simulink model "model"  (R2025b)
settings: Solver=FixedStepDiscrete  StartTime=0.0  StopTime=620  FixedStep=deltaT  RelTol=1e-3
values from neighbouring files (symbols this model uses):
  DegreeToRadian = pi/180    (= 0.0174532925199)    [main8.m]    (also in modelRunner.m)
  g = 9.81    [main8.m]    (also in modelRunner.m)
  Mass = 1.3    [main8.m]    (also in modelRunner.m)
  R_phi = place(A_phi, B_phi, poles_phi)    [main8.m]    (also in modelRunner.m)
  R_psi = place(A_psi, B_psi, poles_psi)    [main8.m]    (also in modelRunner.m)
  R_theta = place(A_theta, B_theta, poles_theta)    [main8.m]    (also in modelRunner.m)
  R_x = place(A_x, B_x, poles_x)    [main8.m]    (also in modelRunner.m)
  R_y = place(A_y, B_y, poles_y)    [main8.m]    (also in modelRunner.m)
  R_z = place(A_z, B_z, poles_z)    [main8.m]    (also in modelRunner.m)
  trajectory_data = TrajectorySetup()    [modelRunner.m]
settings Model: Creator=kuba  LastModifiedBy=kuba

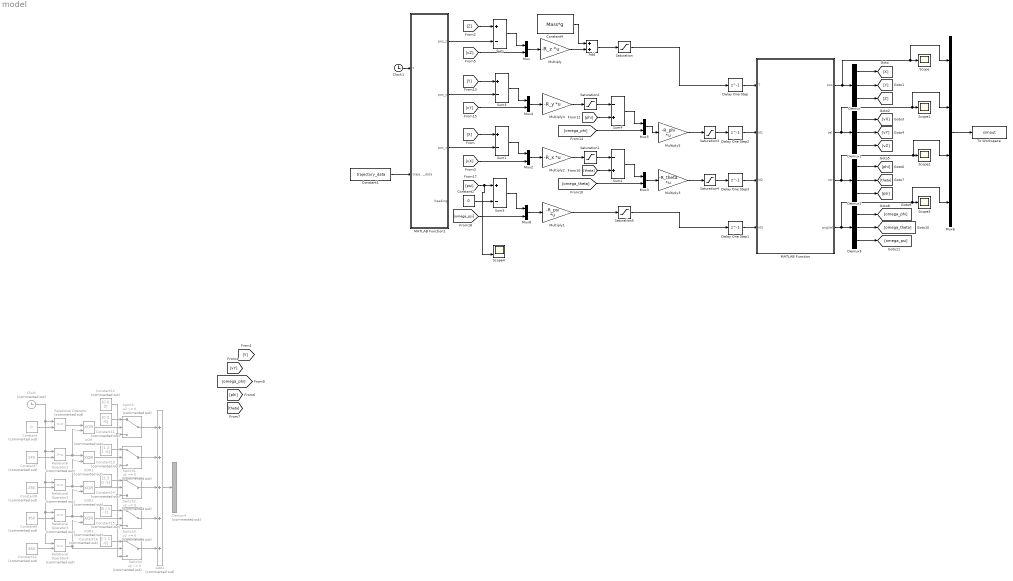
== system model ==
  Add : Sum
  Add1 : Sum  Commented=on  Inputs=+++++
  Clock : Clock  Commented=on
  Clock1 : Clock
  Constant : Constant  Commented=on  Value=0
  Constant1 : Constant  Value=trajectory_data  OutDataTypeStr=Bus: trajectory_data_bus
  Constant10 : Constant  Commented=on  Value=480
  Constant11 : Constant  Commented=on  Value=[0 0 -6]
  Constant12 : Constant  Commented=on  Value=[0 0 0]
  Constant13 : Constant  Commented=on  Value=[1.2 1 -6]
  Constant14 : Constant  Commented=on  Value=[1.5 0 -5]
  Constant15 : Constant  Commented=on  Value=[0 1.5 -7]
  Constant16 : Constant  Commented=on  Value=[-1 1 -6]
  Constant2 : Constant  Value=0
  Constant4 : Constant  Value=Mass*g
  Constant7 : Constant  Commented=on  Value=140
  Constant8 : Constant  Commented=on  Value=280
  Constant9 : Constant  Commented=on  Value=360
  Delay One Step{,1..3} (4 alike) : Delay  DelayLength=1
  Demux{,1..3} (4 alike) : Demux  Outputs=3
  Demux4 : Demux  Commented=on  Outputs=3
  MATLAB Function : MATLAB Function  TreatAsAtomicUnit=on
  MATLAB Function1 : MATLAB Function  TreatAsAtomicUnit=on
  Multiply : Gain  Gain=-R_z  Multiplication=Matrix(K*u)
  Multiply1 : Gain  Gain=-R_psi  Multiplication=Matrix(K*u)
  Multiply2 : Gain  Gain=-R_x  Multiplication=Matrix(K*u)
  Multiply3 : Gain  Gain=-R_theta  Multiplication=Matrix(K*u)
  Multiply4 : Gain  Gain=-R_y  Multiplication=Matrix(K*u)
  Multiply5 : Gain  Gain=-R_phi  Multiplication=Matrix(K*u)
  Mux{,2..5,8} (6 alike) : Mux  Inputs=2
  Mux6 : Mux
  Relational Operator{,1..4} (5 alike) : RelationalOperator  Commented=on  OutDataTypeStr=boolean  RndMeth=Simplest  InputSameDT=off
  Saturation : Saturate  UpperLimit=2*Mass*g  LowerLimit=0
  Saturation1 : Saturate  UpperLimit=10*DegreeToRadian  LowerLimit=-10*DegreeToRadian
  Saturation2 : Saturate  UpperLimit=10*DegreeToRadian  LowerLimit=-10*DegreeToRadian
  Saturation3 : Saturate
  Saturation4 : Saturate
  Saturation5 : Saturate
  Scope{,1..3} (4 alike) : Scope
      Scope settings: ActiveDisplayYMinimum=-8  ActiveDisplayYMaximum=4
      Scope1 settings: ActiveDisplayYMinimum=-1  ActiveDisplayYMaximum=1
      Scope2 settings: ActiveDisplayYMinimum=-2.2668626581836264  ActiveDisplayYMaximum=1.3525904192916169  DataLoggingVariableName=ScopeData2
      Scope3 settings: ActiveDisplayYMinimum=-2.2668626581836264  ActiveDisplayYMaximum=1.3525904192916169  DataLoggingVariableName=ScopeData3
  Scope4 : Scope  NumInputPorts=2
      settings: ActiveDisplayYMinimum=-3.9260838367625022  ActiveDisplayYMaximum=3.9229316294067531  DataLoggingVariableName=ScopeData4
  Sum{,1,3,5} (4 alike) : Sum  Inputs=+-
  Sum2 : Sum  Inputs=-+
  Sum4 : Sum  Inputs=-+
  Switch{,1..4} (5 alike) : Switch  Commented=on  Criteria=u2 ~= 0  SaturateOnIntegerOverflow=off  InputSameDT=off
  To Workspace : ToWorkspace  VariableName=simout  SaveFormat=Timeseries  SampleTime=-1
  XOR{,1..3} (4 alike) : Logic  Commented=on  Operator=XOR  IconShape=distinctive  AllPortsSameDT=off  OutDataTypeStr=boolean
  wires:
  Demux/1 -> [X]
  Demux/2 -> [Y]
  Demux/3 -> [Z]
  Demux1/1 -> [vX]
  Demux1/2 -> [vY]
  Demux1/3 -> [vZ]
  Demux2/1 -> [phi]
  Demux2/2 -> [theta]
  Demux2/3 -> [psi]
  Demux3/1 -> [omega_phi]
  Demux3/2 -> [omega_theta]
  Demux3/3 -> [omega_psi]
  [Z] -> Sum/1
  [vZ] -> Mux/2
  Sum/1 -> Mux/1
  Mux/1 -> Multiply/1
  Multiply/1 -> Add/2
  Constant4/1 -> Add/1
  Multiply3/1 -> Saturation4/1
  Multiply5/1 -> Saturation3/1
  Add/1 -> Saturation/1
  MATLAB Function/4(angVel) -> Mux6/4, Scope3/1, Demux3/1
  MATLAB Function/3(rot) -> Mux6/3, Scope2/1, Demux2/1
  MATLAB Function/2(vel) -> Mux6/2, Scope1/1, Demux1/1
  Delay One Step/1 -> MATLAB Function/1(T)
  MATLAB Function/1(pos) -> Mux6/1, Scope/1, Demux/1
  Multiply1/1 -> Saturation5/1
  Delay One Step1/1 -> MATLAB Function/4(M3)
  Sum1/1 -> Mux2/1
  Mux2/1 -> Multiply2/1
  [vX] -> Mux2/2
  [X] -> Sum1/1
  Multiply2/1 -> Saturation1/1
  Saturation1/1 -> Sum2/1
  Mux3/1 -> Multiply3/1
  [omega_theta] -> Mux3/2
  [theta] -> Sum2/2
  Sum2/1 -> Mux3/1
  Multiply4/1 -> Saturation2/1
  Sum4/1 -> Mux5/1
  Mux4/1 -> Multiply4/1
  [phi] -> Sum4/2
  [vY] -> Mux4/2
  Saturation2/1 -> Sum4/1
  Mux5/1 -> Multiply5/1
  Sum3/1 -> Mux4/1
  [omega_phi] -> Mux5/2
  [Y] -> Sum3/1
  Delay One Step2/1 -> MATLAB Function/2(M1)
  Delay One Step3/1 -> MATLAB Function/3(M2)
  Constant/1 -> Relational Operator/2
  Constant7/1 -> Relational Operator1/2
  Constant8/1 -> Relational Operator2/2
  Constant9/1 -> Relational Operator3/2
  Clock/1 -> Relational Operator4/1, Relational Operator3/1, Relational Operator2/1, Relational Operator1/1, Relational Operator/1
  Constant10/1 -> Relational Operator4/2
  Constant11/1 -> Switch/1
  Constant13/1 -> Switch1/1
  Constant14/1 -> Switch2/1
  Constant15/1 -> Switch3/1
  Constant12/1 -> Switch4/3, Switch3/3, Switch2/3, Switch1/3, Switch/3
  Constant16/1 -> Switch4/1
  Relational Operator/1 -> XOR/1
  XOR/1 -> Switch/2
  Relational Operator2/1 -> XOR1/2, XOR2/1
  Relational Operator1/1 -> XOR1/1, XOR/2
  XOR1/1 -> Switch1/2
  Relational Operator3/1 -> XOR2/2, XOR3/1
  XOR2/1 -> Switch2/2
  Relational Operator4/1 -> Switch4/2, XOR3/2
  XOR3/1 -> Switch3/2
  Switch/1 -> Add1/1
  Switch1/1 -> Add1/2
  Switch2/1 -> Add1/3
  Switch3/1 -> Add1/4
  Switch4/1 -> Add1/5
  Add1/1 -> Demux4/1
  Saturation3/1 -> Delay One Step2/1
  Saturation4/1 -> Delay One Step3/1
  Saturation5/1 -> Delay One Step1/1
  Saturation/1 -> Delay One Step/1
  Clock1/1 -> MATLAB Function1/1(t)
  MATLAB Function1/3(pos_x) -> Sum1/2
  MATLAB Function1/2(pos_y) -> Sum3/2
  MATLAB Function1/1(pos_z) -> Sum/2
  Constant1/1 -> MATLAB Function1/2(trajectory_data)
  Mux6/1 -> To Workspace/1
  [psi] -> Scope4/2, Sum5/1
  [omega_psi] -> Mux8/2
  Sum5/1 -> Mux8/1
  Mux8/1 -> Multiply1/1
  Constant2/1 -> Sum5/2

== matlab function model/MATLAB Function1 ==
  data: pos_z output; pos_y output; t input; pos_x output; trajectory_data input; heading output
function [pos_z, pos_y, pos_x, heading] = TrajectoryReference(t, trajectory_data)
% vel_x, vel_y, vel_z, acc_x, acc_y, acc_z, heading, speed
    % TrajectoryReference - Trajectory lookup for quadcopter waypoint tracking
    %
    % Usage in Simulink:
    %   [pos_x, pos_y, pos_z, vel_x, vel_y, vel_z, acc_x, acc_y, acc_z, heading, speed] = TrajectoryReference(t, trajectory_data)
    %
    % Inputs:
    %   t - current simulation time [s]
    %   trajectory_data - structure containing pre-computed trajectory (from TrajectorySetup.m)
    %
    % Outputs:
    %   pos_x, pos_y, pos_z - desired position [m]
    %   vel_x, vel_y, vel_z - desired velocity [m/s]
    %   acc_x, acc_y, acc_z - desired acceleration [m/s^2]
    %   heading - desired yaw angle [rad]
    %   speed - total velocity magnitude [m/s]
    
    % Clamp time to valid trajectory range
    t_clamped = max(trajectory_data.t_min, min(t, trajectory_data.t_max));
    
    % Linear interpolation on the pre-computed grid
    pos_x = interp1(trajectory_data.time, trajectory_data.pos_x, t_clamped, 'linear');
    pos_y = interp1(trajectory_data.time, trajectory_data.pos_y, t_clamped, 'linear');
    pos_z = interp1(trajectory_data.time, trajectory_data.pos_z, t_clamped, 'linear');
    
    vel_x = interp1(trajectory_data.time, trajectory_data.vel_x, t_clamped, 'linear');
    vel_y = interp1(trajectory_data.time, trajectory_data.vel_y, t_clamped, 'linear');
    vel_z = interp1(trajectory_data.time, trajectory_data.vel_z, t_clamped, 'linear');
    
    acc_x = interp1(trajectory_data.time, trajectory_data.acc_x, t_clamped, 'linear');
    acc_y = interp1(trajectory_data.time, trajectory_data.acc_y, t_clamped, 'linear');
    acc_z = interp1(trajectory_data.time, trajectory_data.acc_z, t_clamped, 'linear');
    
    heading = interp1(trajectory_data.time, trajectory_data.heading, t_clamped, 'linear');
    speed = interp1(trajectory_data.time, trajectory_data.speed, t_clamped, 'linear');
end

== matlab function model/MATLAB Function ==
  data: T input; pos output; M1 input; M2 input; M3 input; vel output; rot output; angVel output
function [pos, vel, rot, angVel] = QuadcopterSimulinkFunction(T, M1, M2, M3)
    % Simulink-compatible quadcopter dynamics function
    % Inputs: E (external forces) T (thrust), M1, M2, M3 (moments)
    % Outputs: pos (3x1), vel (3x1), rot (3x1 Euler angles), angVel (3x1)
    
    persistent state initialized mass I_matrix g dt
    
    % Initialize on first call
    if isempty(initialized)
        % Physical parameters
        mass = 1.3;
        I_matrix = [0.023 0 0; 0 0.023 0; 0 0 0.047];
        g = 9.81;
        dt = 0.1;  % Simulation time step
        
        % State vector: [pos(3), vel(3), euler(3), angVel(3)]
        state = zeros(12, 1);
        state(3) = 0;  % Initial z position (ground level)
        
        initialized = true;
    end
    
    % Extract state components
    pos_x = state(1);
    pos_y = state(2);
    pos_z = state(3);
    vel_x = state(4);
    vel_y = state(5);
    vel_z = state(6);
    phi = state(7);
    theta = state(8);
    psi = state(9);
    dPhi = state(10);
    dTheta = state(11);
    dPsi = state(12);
    
    % Rotation matrix from Euler angles (body to inertial)
    Rphi = [1 0 0; 0 cos(phi) -sin(phi); 0 sin(phi) cos(phi)];
    Rtheta = [cos(theta) 0 sin(theta); 0 1 0; -sin(theta) 0 cos(theta)];
    Rpsi = [cos(psi) -sin(psi) 0; sin(psi) cos(psi) 0; 0 0 1];
    R = Rpsi * Rtheta * Rphi;
    
    % Position derivatives
    dPos = [vel_x; vel_y; vel_z];
    
    % Velocity derivatives (acceleration)
    % a = (1/m) * (R * [0; 0; -T] + [0; 0; mg])

    if (pos_z == 0)
        T = max(T, mass * g);
    end

    gravity = [0; 0; g * mass];

    thrust_body = [0; 0; -T];
    thrust_inertial = R * thrust_body;
    dVel = (1 / mass) * (gravity + thrust_inertial);
    
    % Euler angle derivatives from angular rates
    dEuler = [1, sin(phi)*tan(theta), cos(phi)*tan(theta);
              0, cos(phi), -sin(phi);
              0, sin(phi)*sec(theta), cos(phi)*sec(theta)] * [dPhi; dTheta; dPsi];
    
    % Angular velocity derivatives from attitude dynamics
    % I * dw = M - w x (I * w)
    w = [dPhi; dTheta; dPsi];
    M = [M1; M2; M3];
    dAngVel = I_matrix \ (M - cross(w, I_matrix * w));
    
    % Assemble full derivative vector
    dState = [dPos; dVel; dEuler; dAngVel];
    
    % Euler integration
    state = state + dState * dt;
    
    % Output current state
    pos = state(1:3);
    vel = state(4:6);
    rot = state(7:9);
    angVel = state(10:12);
end
